simulink model "LAB_2_GROUP_1_ASS_1"  (R2019a)
settings: Solver=VariableStepAuto  StartTime=0.0  StopTime=10.0  RelTol=1e-3
libraries: simulink x1
settings Model: Creator=fiado  LastModifiedBy=fiado

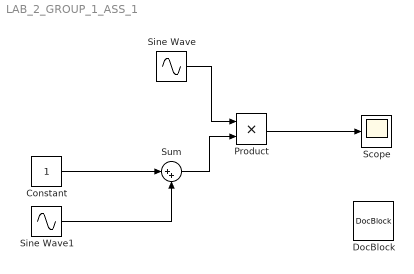
== system LAB_2_GROUP_1_ASS_1 ==
  Constant : Constant
  DocBlock : simulink/Model-Wide Utilities/DocBlock  DocumentType=Text
      content=|
      | Type your documentation hereAmplitude Modulation (AM) with a tone modulator having a unity modulation index is expressed as:
      | x(t) = (1 + cos(t)) * cos(2t)
      |
      | Simulation Details:
      | - Simulation Time: 10 seconds
      |
      | Description:
      | This Simulink model demonstrates Amplitude Modulation (AM) with a unity modulation index. The input signal is a cosine wave, and it is modulated with the (1 + cos(t)) signal. The resulting AM signal x(t) is obtained by multiplying the modulating signal with the carrier signal.
      |
      | Model Overview:
      | - The "Sine Wave 1" block generates the cosine wave (cos(t)).
      | - The "Sine Wave" block generates the carrier signal (cos(2t)).
      | - The "Add" block combines the modulating signal (cos(t)) and the constant 1.
      | - The "Product" block combines the result from the add block with the carrier signal (cos(2t))
      | - The "Scope" block displays the AM signal x(t).
      | - Simulation time is set to 10 seconds for observing the complete waveform.
  Product : Product
  Scope : Scope
  Sine Wave : Sin  Frequency=0.318  Phase=90  SampleTime=0
  Sine Wave1 : Sin  Frequency=0.159  Phase=90  SampleTime=0
  Sum : Sum  Inputs=|++
  wires:
  Constant/1 -> Sum/1
  Sine Wave1/1 -> Sum/2
  Product/1 -> Scope/1
  Sine Wave/1 -> Product/1
  Sum/1 -> Product/2
